simulink model "ver5_mck_system"  (R2017b)
settings: Solver=FixedStepAuto  StartTime=0.0  StopTime=100  FixedStep=10e-5  RelTol=1e-3
InitFcn:
  | ver5_mck
values from neighbouring files (symbols this model uses):
  A_new = [A,zeros(2,1) ... (first row only)    [ver5_mck.m]
  B_new = [B ... (first row only)    [ver5_mck.m]
  E = [0 ... (first row only)    [ver5_mck.m]
  K = place(A,B,p)    [LinearizedPendulumModel.m]    (also in ver5_mck.m = dlqr(A_new,B_new,Q,R))
  Ts = 0.01    [ver5_mck.m]
settings Model: Creator=Mehmet  LastModifiedBy=Mehmet

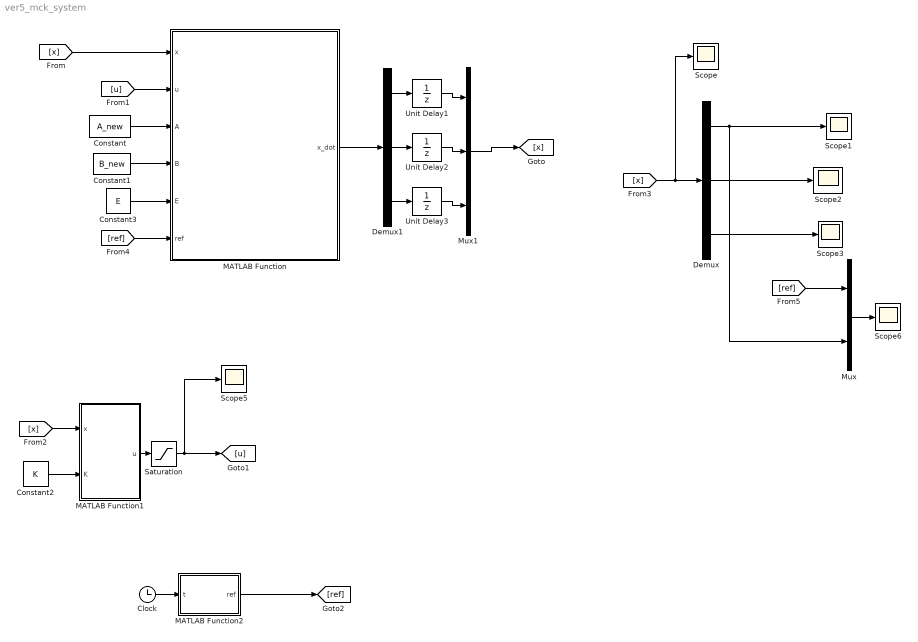
== system ver5_mck_system ==
  Clock : Clock
  Constant : Constant  Value=A_new  VectorParams1D=off
  Constant1 : Constant  Value=B_new  VectorParams1D=off
  Constant2 : Constant  Value=K  VectorParams1D=off
  Constant3 : Constant  Value=E  VectorParams1D=off
  Demux : Demux  Outputs=3
  Demux1 : Demux  Outputs=3
  MATLAB Function : MATLAB Function  TreatAsAtomicUnit=on
  MATLAB Function1 : MATLAB Function  TreatAsAtomicUnit=on
  MATLAB Function2 : MATLAB Function  TreatAsAtomicUnit=on
  Mux : Mux  Inputs=2
  Mux1 : Mux  Inputs=3
  Saturation : Saturate  UpperLimit=100  LowerLimit=-100
  Scope{,1..3,5..6} (6 alike) : Scope
  Unit Delay1 : UnitDelay  SampleTime=Ts*4
  Unit Delay2 : UnitDelay  SampleTime=Ts/4
  Unit Delay3 : UnitDelay  SampleTime=Ts/5
  wires:
  Demux/2 -> Scope2/1
  Constant3/1 -> MATLAB Function/5(E)
  Mux/1 -> Scope6/1
  [u] -> MATLAB Function/2(u)
  Demux/3 -> Scope3/1
  [ref] -> Mux/1
  Constant1/1 -> MATLAB Function/4(B)
  [x] -> MATLAB Function/1(x)
  Constant/1 -> MATLAB Function/3(A)
  [x] -> Scope/1, Demux/1
  Demux/1 -> Mux/2, Scope1/1
  [ref] -> MATLAB Function/6(ref)
  MATLAB Function1/1(u) -> Saturation/1
  Constant2/1 -> MATLAB Function1/2(K)
  Saturation/1 -> Scope5/1, [u]
  MATLAB Function2/1(ref) -> [ref]
  [x] -> MATLAB Function1/1(x)
  Clock/1 -> MATLAB Function2/1(t)
  MATLAB Function/1(x_dot) -> Demux1/1
  Demux1/1 -> Unit Delay1/1
  Demux1/2 -> Unit Delay2/1
  Demux1/3 -> Unit Delay3/1
  Unit Delay1/1 -> Mux1/1
  Unit Delay2/1 -> Mux1/2
  Unit Delay3/1 -> Mux1/3
  Mux1/1 -> [x]

== matlab function ver5_mck_system/MATLAB Function1 ==
  data: x input; u output; K input
function u = fcn(x,K)

u = -K*x;

end

== matlab function ver5_mck_system/MATLAB Function ==
  data: x input; u input; x_dot output; A input; B input; E input; ref input
function x_dot = fcn(x,u,A,B,E,ref)

x_new = zeros(3,1);

x_new = x;

% output
x_dot = A*x_new + B*u + E*ref;

end

== matlab function ver5_mck_system/MATLAB Function2 ==
  data: t input; ref output
function ref = fcn(t)


f = 0.2;

A = 1;
B = 5;

ref = A*sin(2*pi*f*t) + B;

end
